simulink model "regulator2"  (R2019a)
settings: Solver=FixedStepAuto  StartTime=0.0  StopTime=10  FixedStep=sT  RelTol=1e-3
InitFcn:
  | param2;
values from neighbouring files (symbols this model uses):
  A = [0 1; w^2 0]    [continus.m]    (also in discrete.m = [0 1; omega^2 0]; param.m = [0 1; omega^2 0]; param2.m = [0 1; omega^2 0]; param_kf.m)
  B = [0; -w^2]    [continus.m]    (also in discrete.m = [0; -omega^2]; param.m = [0; -omega^2]; param2.m = [0; -omega^2]; param_kf.m)
  C = eye(2)    [discrete.m]    (also in param.m; param2.m; param_kf.m = [w^2 0]; test0.m)
  D = [0 0]'    [discrete.m]    (also in param.m; param2.m; param_kf.m = -w^2; test0.m)
  inix = [0.00 0.0]'    [param.m]    (also in param2.m = [0.05 0.0]'; param_kf.m = [0.0 0.0]')
  K = [k1 k2]    [continus.m]    (also in discrete.m = -place(A, B, [q1 q2]); param.m; param2.m = dlqr(A,B,Q,H); param_kf.m = -place(A, B, [q1 q2]))
  sT = 0.01    [discrete.m]    (also in param.m; param2.m; param_kf.m; test0.m)
settings Model: Creator=hideaki  LastModifiedBy=hideaki

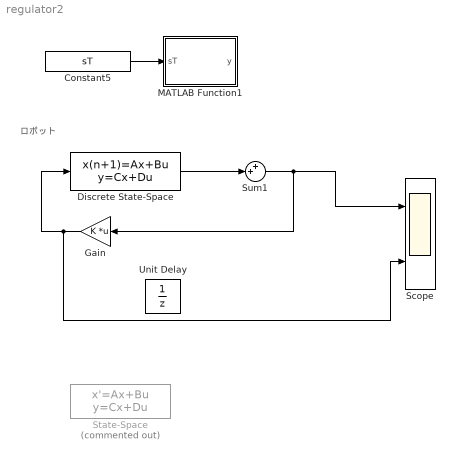
== system regulator2 ==
  note: ロボット
  Constant5 : Constant  Value=sT
  Discrete State-Space : DiscreteStateSpace  A=A  B=B  C=C  D=D  InitialCondition=inix  SampleTime=sT
  Gain : Gain  Gain=K  Multiplication=Matrix(K*u)
  MATLAB Function1 : MATLAB Function  TreatAsAtomicUnit=on  SystemSampleTime=sT
  Scope : Scope  NumInputPorts=2
  State-Space : StateSpace  Commented=on  A=A  B=B  C=C  D=D  InitialCondition=inix
  Sum1 : Sum  Inputs=++|
  Unit Delay : UnitDelay  SampleTime=-1  HasFrameUpgradeWarning=on
  wires:
  Discrete State-Space/1 -> Sum1/2
  Gain/1 -> Discrete State-Space/1, Scope/2
  Constant5/1 -> MATLAB Function1/1(sT)
  Sum1/1 -> Gain/1, Scope/1

== matlab function regulator2/MATLAB Function1 ==
  data: y output; sT input
function y = nois(sT)
    
    y = zeros(2,1);
    persistent tCnt;
    if isempty(tCnt)
        tCnt = 0;
    end
    
    if (tCnt >= 1 && tCnt <= 1.06) 
        y(2) = -0.3;
    end
    
    tCnt = tCnt + sT;
end
